simulink model "model_chirp_control_conMR_BoucWen"  (R2021b)
settings: Solver=VariableStepAuto  StartTime=0.0  StopTime=t_final2  FixedStep=tsam  RelTol=1e-3  EnableMultiTasking=on
values from neighbouring files (symbols this model uses):
  A = [      0          1       0    0      0    0 ... (first row only)    [model.m]
  I1 = 0.01    [Run_MdE_Research_Report_con_MR_damper.m]
  kt = ((2*pi*ft)^2)*mt    [Run_MdE_Research_Report.m]    (also in Run_MdE_Research_Report_con_MR_damper.m; my_script.m)
  mt = mu*m1    (= 0.02)    [Run_MdE_Research_Report.m]    (also in Run_MdE_Research_Report_con_MR_damper.m = 40; my_script.m)
undefined symbols (not defined in the file or in its folder): B, C, D_Gs, k0, N_Gs, ndata2, t_final2, tsam, x0
libraries: simulink x1
settings Model: Creator=user  LastModifiedBy=luismiguelmartinezgomez
settings SolverCC: AlgebraicLoopSolver=TrustRegion
settings DataIOCC: LimitDataPoints=on  SaveFormat=Array  SignalLoggingSaveFormat=ModelDataLogs  ReturnWorkspaceOutputs=off  SignalLoggingName=sigsOut
settings OptimizationCC: InitFltsAndDblsToZero=on  LifeSpan=inf
settings DebuggingCC: SaveWithParameterizedLinksMsg=none  UnderspecifiedInitializationDetection=Classic  MergeDetectMultiDrivingBlocksExec=none  SignalResolutionControl=TryResolveAllWithWarning  MultiTaskDSMMsg=warning  MultiTaskCondExecSysMsg=none  FcnCallInpInsideContextMsg=warning  SFUnexpectedBacktrackingDiag=warning  SFNoUnconditionalDefaultTransitionDiag=warning  SFMachineParentedDataDiag=warning  ArithmeticOperatorsInVariantConditions=warning
settings HardwareCC: ProdBitPerPointer=32  ProdBitPerSizeT=32  ProdBitPerPtrDiffT=32  ProdLargestAtomicFloat=None  ProdIntDivRoundTo=Undefined  ProdEndianess=Unspecified  ProdWordSize=32  ProdHWDeviceType=32-bit Generic  TargetBitPerLong=64  TargetBitPerPointer=64  TargetBitPerSizeT=64  TargetBitPerPtrDiffT=64  TargetLongLongMode=on  TargetIntDivRoundTo=Zero  TargetEndianess=LittleEndian  TargetWordSize=64  TargetHWDeviceType=MATLAB Host  ProdEqTarget=off
settings ModelReferenceCC: PropagateSignalLabelsOutOfModel=off
settings SFSimCC: SimUseLocalCustomCode=off  CustomCodeUndefinedFunction=UseInterfaceOnly
settings RTWCC: RTWUseLocalCustomCode=off
settings CodeAppCC: StateflowObjectComments=on
settings GRTTargetCC: TargetFcnLib=ansi_tfl_tmw.mat  TargetLangStandard=C89/C90 (ANSI)  CombineOutputUpdateFcns=off  GRTInterface=on
settings ConfigComp: CovMetricSettings=dw  CovSaveCumulativeToWorkspaceVar=on  CovSaveSingleToWorkspaceVar=on  CovExternalEMLEnable=off  CovSFcnEnable=off

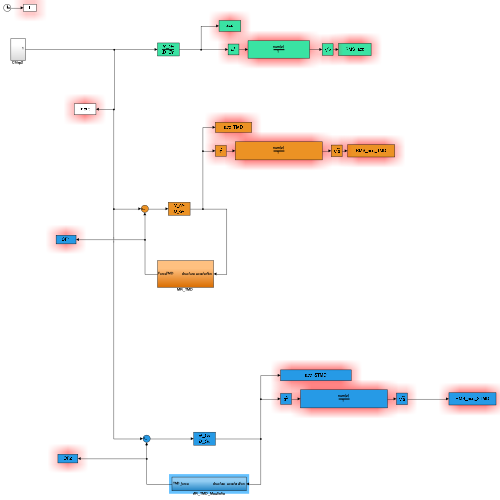
[thumbnail: Simulink's stored preview of the top-level diagram]
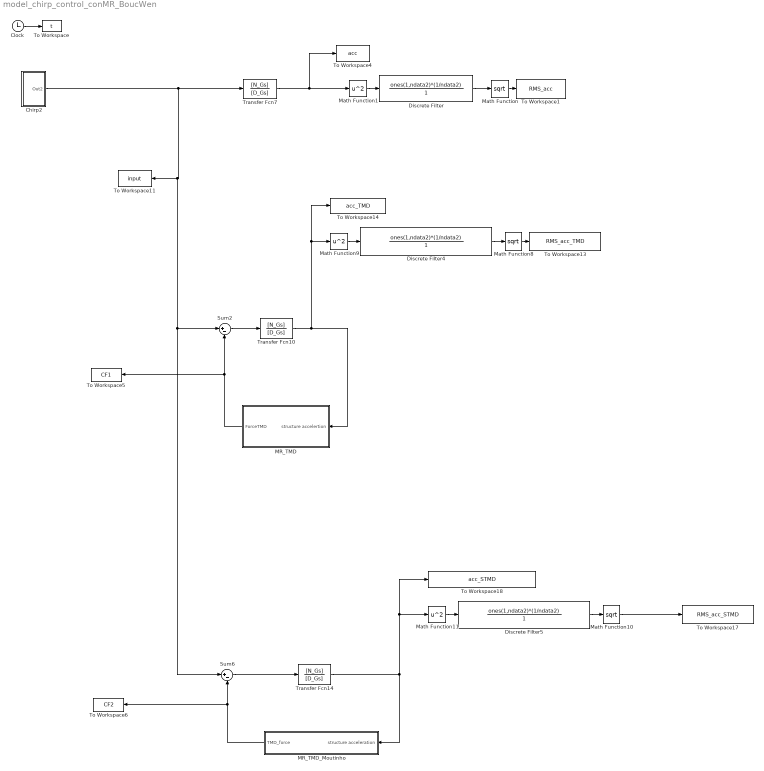
== system model_chirp_control_conMR_BoucWen ==
  Chirp2 : Subsystem
  Clock : Clock
  Discrete Filter : DiscreteFilter  Numerator=ones(1,ndata2)*(1/ndata2)  Denominator=1  SampleTime=tsam
  Discrete Filter4 : DiscreteFilter  Numerator=ones(1,ndata2)*(1/ndata2)  Denominator=1  SampleTime=tsam
  Discrete Filter5 : DiscreteFilter  Numerator=ones(1,ndata2)*(1/ndata2)  Denominator=1  SampleTime=tsam
  MR_TMD : Subsystem
  MR_TMD_Moutinho : Subsystem
  Math Function : Math  Operator=sqrt  SignedPower=on  SampleTime=tsam  SaturateOnIntegerOverflow=on
  Math Function1 : Math  Operator=square  SignedPower=on  SampleTime=tsam  SaturateOnIntegerOverflow=on
  Math Function10 : Math  Operator=sqrt  SignedPower=on  SampleTime=tsam  SaturateOnIntegerOverflow=on
  Math Function11 : Math  Operator=square  SignedPower=on  SampleTime=tsam  SaturateOnIntegerOverflow=on
  Math Function8 : Math  Operator=sqrt  SignedPower=on  SampleTime=tsam  SaturateOnIntegerOverflow=on
  Math Function9 : Math  Operator=square  SignedPower=on  SampleTime=tsam  SaturateOnIntegerOverflow=on
  Sum2 : Sum  Inputs=|+-
  Sum6 : Sum  Inputs=|+-
  To Workspace : ToWorkspace  VariableName=t  SampleTime=tsam
  To Workspace1 : ToWorkspace  VariableName=RMS_acc  SampleTime=tsam
  To Workspace11 : ToWorkspace  VariableName=input  SampleTime=tsam
  To Workspace13 : ToWorkspace  VariableName=RMS_acc_TMD  SampleTime=tsam
  To Workspace14 : ToWorkspace  VariableName=acc_TMD  SampleTime=tsam
  To Workspace17 : ToWorkspace  VariableName=RMS_acc_STMD  SampleTime=tsam
  To Workspace18 : ToWorkspace  VariableName=acc_STMD  SampleTime=tsam
  To Workspace4 : ToWorkspace  VariableName=acc  SampleTime=tsam
  To Workspace5 : ToWorkspace  VariableName=CF1  SampleTime=tsam
  To Workspace6 : ToWorkspace  VariableName=CF2  SampleTime=tsam
  Transfer Fcn10 : TransferFcn  Numerator=[N_Gs]  Denominator=[D_Gs]
  Transfer Fcn14 : TransferFcn  Numerator=[N_Gs]  Denominator=[D_Gs]
  Transfer Fcn7 : TransferFcn  Numerator=[N_Gs]  Denominator=[D_Gs]
  wires:
  Clock/1 -> To Workspace/1
  Math Function1/1 -> Discrete Filter/1
  Discrete Filter/1 -> Math Function/1
  Math Function/1 -> To Workspace1/1
  Sum2/1 -> Transfer Fcn10/1
  Math Function9/1 -> Discrete Filter4/1
  Discrete Filter4/1 -> Math Function8/1
  Math Function8/1 -> To Workspace13/1
  MR_TMD/1(ForceTMD) -> Sum2/2, To Workspace5/1
  Transfer Fcn7/1 -> Math Function1/1, To Workspace4/1
  Transfer Fcn10/1 -> MR_TMD/1(structure accelertion), To Workspace14/1, Math Function9/1
  Math Function11/1 -> Discrete Filter5/1
  Discrete Filter5/1 -> Math Function10/1
  Math Function10/1 -> To Workspace17/1
  Sum6/1 -> Transfer Fcn14/1
  Chirp2/1(Out2) -> Sum2/1, Sum6/1, To Workspace11/1, Transfer Fcn7/1
  Transfer Fcn14/1 -> MR_TMD_Moutinho/1(structure acceleration), Math Function11/1, To Workspace18/1
  MR_TMD_Moutinho/1(TMD_force) -> To Workspace6/1, Sum6/2

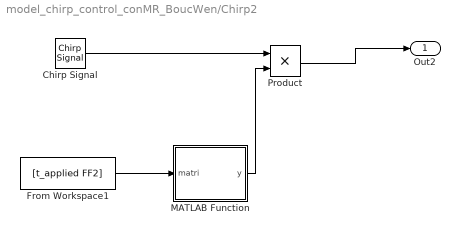
== system model_chirp_control_conMR_BoucWen/Chirp2 ==
  Chirp Signal : simulink/Sources/Chirp Signal  f1=f_ini  T=t_final2  f2=f_fin
  From Workspace1 : FromWorkspace  VariableName=[t_applied FF2]  SampleTime=tsam  ZeroCross=off
  MATLAB Function : MATLAB Function  TreatAsAtomicUnit=on
  Product : Product
  Out2 : Outport
  wires:
  Chirp Signal/1 -> Product/1
  MATLAB Function/1(y) -> Product/2
  Product/1 -> Out2/1
  From Workspace1/1 -> MATLAB Function/1(matri)

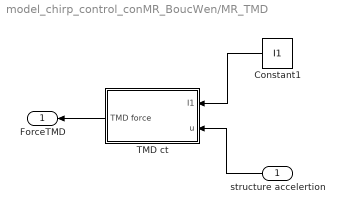
== system model_chirp_control_conMR_BoucWen/MR_TMD ==
  structure accelertion : Inport
  Constant1 : Constant  Value=I1
  TMD ct : Subsystem
  ForceTMD : Outport
  wires:
  TMD ct/1(TMD force) -> ForceTMD/1
  structure accelertion/1 -> TMD ct/2(u)
  Constant1/1 -> TMD ct/1(I1)

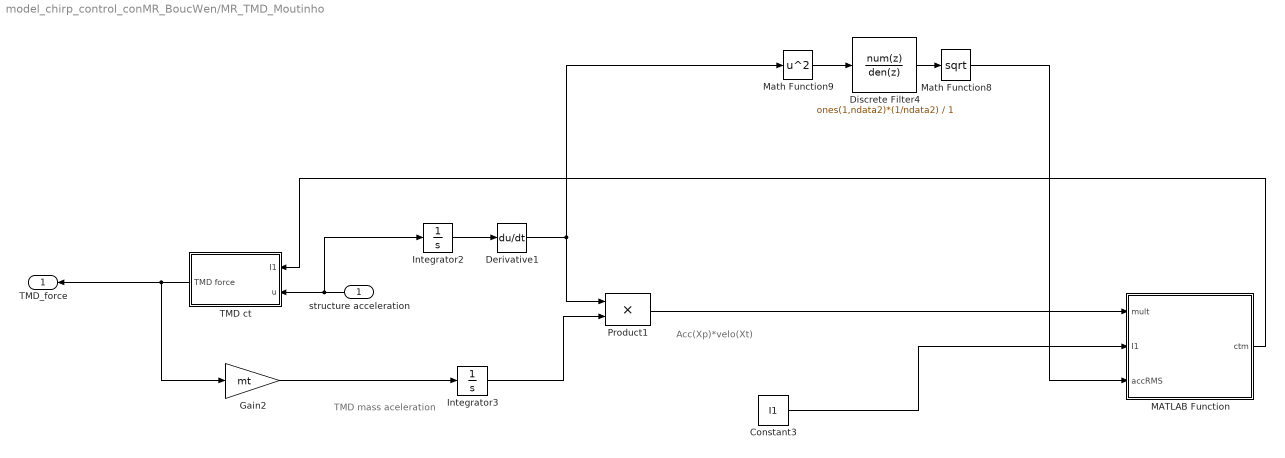
== system model_chirp_control_conMR_BoucWen/MR_TMD_Moutinho ==
  note: TMD mass
      | aceleration
  note: Acc(Xp)*velo(Xt)
  structure acceleration : Inport
  Constant3 : Constant  Value=I1
  Derivative1 : Derivative
  Discrete Filter4 : DiscreteFilter  Numerator=ones(1,ndata2)*(1/ndata2)  Denominator=1  SampleTime=tsam
  Gain2 : Gain  Gain=mt
  Integrator2 : Integrator
  Integrator3 : Integrator
  MATLAB Function : MATLAB Function  TreatAsAtomicUnit=on
  Math Function8 : Math  Operator=sqrt  SignedPower=on  SampleTime=tsam  SaturateOnIntegerOverflow=on
  Math Function9 : Math  Operator=square  SignedPower=on  SampleTime=tsam  SaturateOnIntegerOverflow=on
  Product1 : Product  OutDataTypeStr=double  SaturateOnIntegerOverflow=on
  TMD ct : Subsystem
  TMD_force : Outport
  wires:
  TMD ct/1(TMD force) -> Gain2/1, TMD_force/1
  Integrator3/1 -> Product1/2
  Product1/1 -> MATLAB Function/1(mult)
  MATLAB Function/1(ctm) -> TMD ct/1(I1)
  structure acceleration/1 -> Integrator2/1, TMD ct/2(u)
  Gain2/1 -> Integrator3/1
  Constant3/1 -> MATLAB Function/2(I1)
  Math Function9/1 -> Discrete Filter4/1
  Discrete Filter4/1 -> Math Function8/1
  Math Function8/1 -> MATLAB Function/3(accRMS)
  Integrator2/1 -> Derivative1/1
  Derivative1/1 -> Product1/1, Math Function9/1

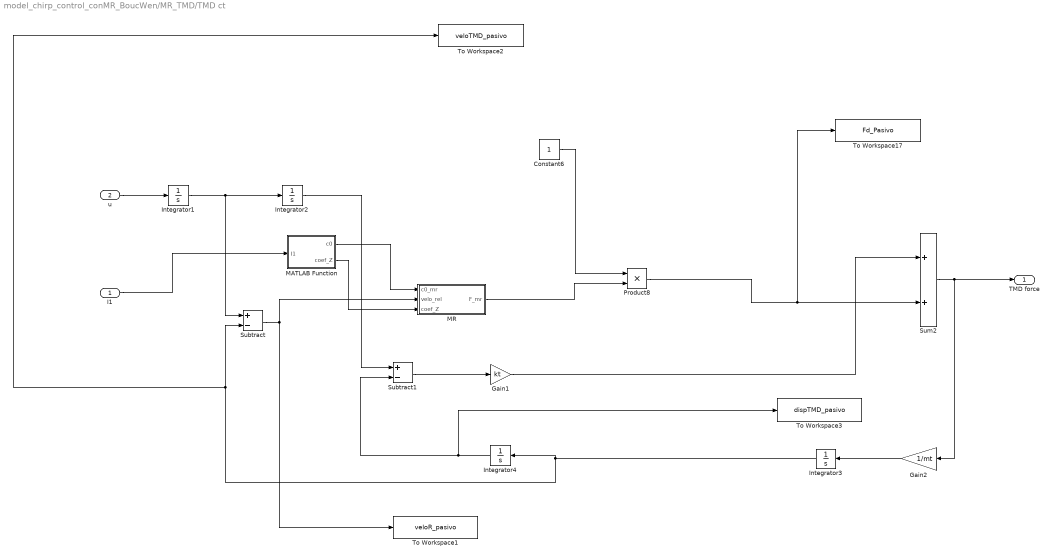
== system model_chirp_control_conMR_BoucWen/MR_TMD/TMD ct ==
  I1 : Inport
  u : Inport  Port=2
  Constant6 : Constant
  Gain1 : Gain  Gain=kt
  Gain2 : Gain  Gain=1/mt
  Integrator{1..4} (4 alike) : Integrator
  MATLAB Function : MATLAB Function  TreatAsAtomicUnit=on
  MR : Subsystem
  Product8 : Product
  Subtract : Sum  Inputs=+-
  Subtract1 : Sum  Inputs=+-
  Sum2 : Sum
  To Workspace1 : ToWorkspace  VariableName=veloR_pasivo  SampleTime=tsam
  To Workspace17 : ToWorkspace  VariableName=Fd_Pasivo  SampleTime=tsam
  To Workspace2 : ToWorkspace  VariableName=veloTMD_pasivo  SampleTime=tsam
  To Workspace3 : ToWorkspace  VariableName=dispTMD_pasivo  SampleTime=tsam
  TMD force : Outport
  wires:
  Integrator1/1 -> Subtract/1, Integrator2/1
  u/1 -> Integrator1/1
  I1/1 -> MATLAB Function/1(I1)
  Integrator3/1 -> Integrator4/1, To Workspace2/1, Subtract/2
  Subtract/1 -> MR/2(velo_rel), To Workspace1/1
  Gain2/1 -> Integrator3/1
  Integrator4/1 -> To Workspace3/1, Subtract1/2
  Integrator2/1 -> Subtract1/1
  Subtract1/1 -> Gain1/1
  Gain1/1 -> Sum2/1
  Sum2/1 -> Gain2/1, TMD force/1
  MATLAB Function/1(c0) -> MR/1(c0_mr)
  MATLAB Function/2(coef_Z) -> MR/3(coef_Z)
  Constant6/1 -> Product8/1
  MR/1(F_mr) -> Product8/2
  Product8/1 -> To Workspace17/1, Sum2/2

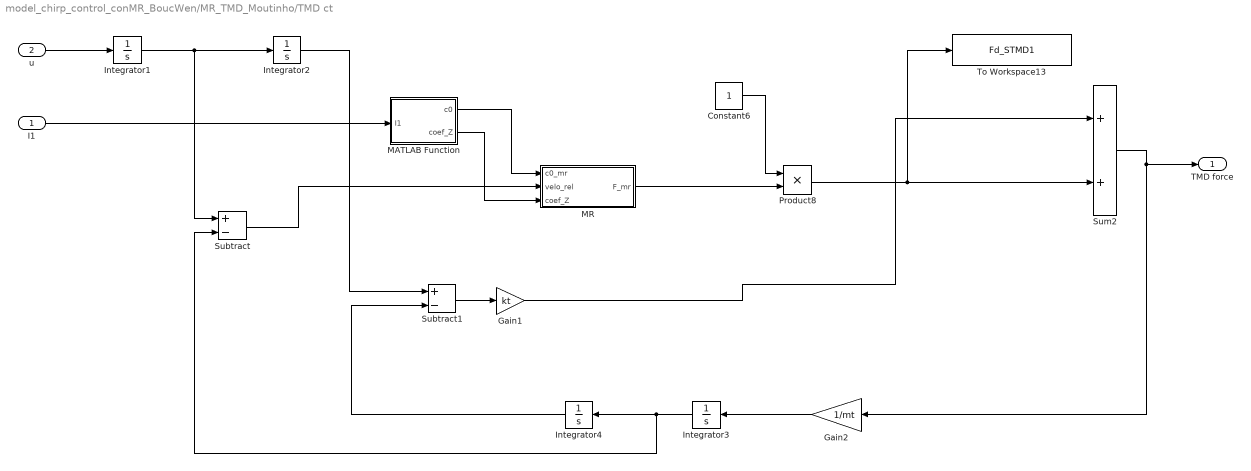
== system model_chirp_control_conMR_BoucWen/MR_TMD_Moutinho/TMD ct ==
  I1 : Inport
  u : Inport  Port=2
  Constant6 : Constant
  Gain1 : Gain  Gain=kt
  Gain2 : Gain  Gain=1/mt
  Integrator{1..4} (4 alike) : Integrator
  MATLAB Function : MATLAB Function  TreatAsAtomicUnit=on
  MR : Subsystem
  Product8 : Product
  Subtract : Sum  Inputs=+-
  Subtract1 : Sum  Inputs=+-
  Sum2 : Sum
  To Workspace13 : ToWorkspace  VariableName=Fd_STMD1  SampleTime=tsam
  TMD force : Outport
  wires:
  Integrator1/1 -> Subtract/1, Integrator2/1
  u/1 -> Integrator1/1
  Integrator3/1 -> Integrator4/1, Subtract/2
  Gain2/1 -> Integrator3/1
  Integrator4/1 -> Subtract1/2
  Integrator2/1 -> Subtract1/1
  Subtract1/1 -> Gain1/1
  Gain1/1 -> Sum2/1
  Sum2/1 -> Gain2/1, TMD force/1
  I1/1 -> MATLAB Function/1(I1)
  Subtract/1 -> MR/2(velo_rel)
  MATLAB Function/1(c0) -> MR/1(c0_mr)
  MATLAB Function/2(coef_Z) -> MR/3(coef_Z)
  Constant6/1 -> Product8/1
  MR/1(F_mr) -> Product8/2
  Product8/1 -> To Workspace13/1, Sum2/2

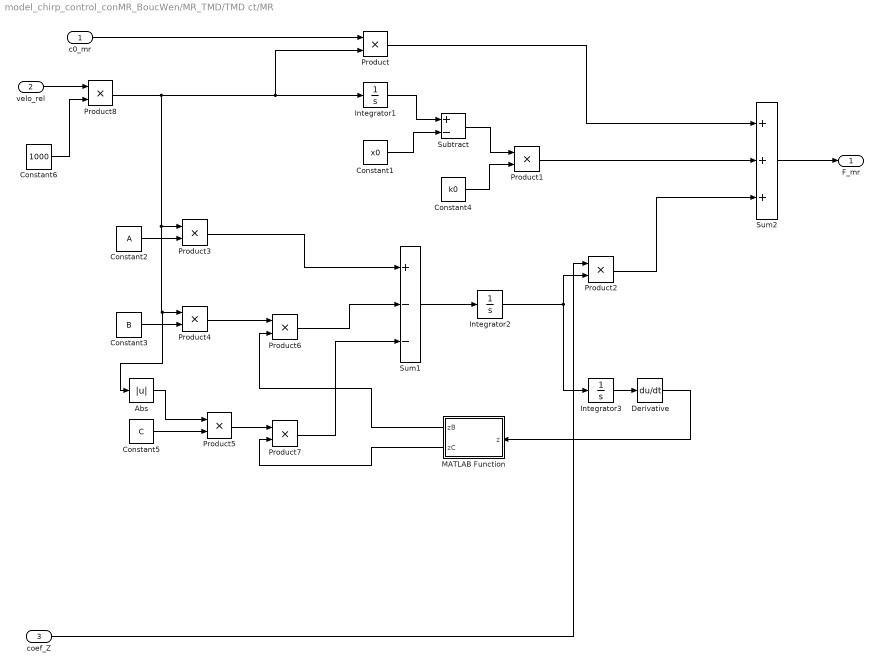
== system model_chirp_control_conMR_BoucWen/MR_TMD/TMD ct/MR ==
  c0_mr : Inport
  velo_rel : Inport  Port=2
  coef_Z : Inport  Port=3
  Abs : Abs
  Constant1 : Constant  Value=x0
  Constant2 : Constant  Value=A
  Constant3 : Constant  Value=B
  Constant4 : Constant  Value=k0
  Constant5 : Constant  Value=C
  Constant6 : Constant  Value=1000
  Derivative : Derivative
  Integrator1 : Integrator
  Integrator2 : Integrator  UpperSaturationLimit=1  LowerSaturationLimit=-1
  Integrator3 : Integrator
  MATLAB Function : MATLAB Function  TreatAsAtomicUnit=on
  Product{,1..8} (9 alike) : Product
  Subtract : Sum  Inputs=+-
  Sum1 : Sum  Inputs=+--
  Sum2 : Sum  Inputs=+++
  F_mr : Outport
  wires:
  c0_mr/1 -> Product/1
  Integrator1/1 -> Subtract/1
  Constant1/1 -> Subtract/2
  Subtract/1 -> Product1/1
  Constant4/1 -> Product1/2
  Sum2/1 -> F_mr/1
  Product1/1 -> Sum2/2
  Product/1 -> Sum2/1
  coef_Z/1 -> Product2/1
  Integrator2/1 -> Integrator3/1, Product2/2
  Constant2/1 -> Product3/2
  Constant3/1 -> Product4/2
  Constant5/1 -> Product5/2
  Sum1/1 -> Integrator2/1
  Product3/1 -> Sum1/1
  Product4/1 -> Product6/1
  Product5/1 -> Product7/1
  MATLAB Function/1(zB) -> Product6/2
  Product6/1 -> Sum1/2
  MATLAB Function/2(zC) -> Product7/2
  Product7/1 -> Sum1/3
  Product2/1 -> Sum2/3
  Integrator3/1 -> Derivative/1
  Derivative/1 -> MATLAB Function/1(z)
  Abs/1 -> Product5/1
  Product8/1 -> Product3/1, Abs/1, Product4/1, Integrator1/1, Product/2
  velo_rel/1 -> Product8/1
  Constant6/1 -> Product8/2

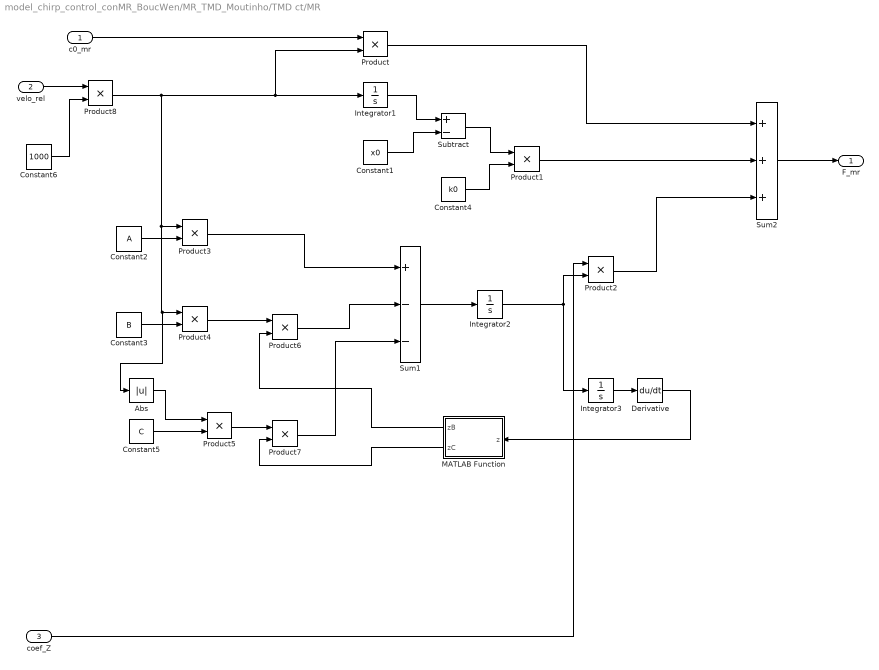
== system model_chirp_control_conMR_BoucWen/MR_TMD_Moutinho/TMD ct/MR ==
  c0_mr : Inport
  velo_rel : Inport  Port=2
  coef_Z : Inport  Port=3
  Abs : Abs
  Constant1 : Constant  Value=x0
  Constant2 : Constant  Value=A
  Constant3 : Constant  Value=B
  Constant4 : Constant  Value=k0
  Constant5 : Constant  Value=C
  Constant6 : Constant  Value=1000
  Derivative : Derivative
  Integrator1 : Integrator
  Integrator2 : Integrator  UpperSaturationLimit=1  LowerSaturationLimit=-1
  Integrator3 : Integrator
  MATLAB Function : MATLAB Function  TreatAsAtomicUnit=on
  Product{,1..8} (9 alike) : Product
  Subtract : Sum  Inputs=+-
  Sum1 : Sum  Inputs=+--
  Sum2 : Sum  Inputs=+++
  F_mr : Outport
  wires:
  c0_mr/1 -> Product/1
  Integrator1/1 -> Subtract/1
  Constant1/1 -> Subtract/2
  Subtract/1 -> Product1/1
  Constant4/1 -> Product1/2
  Sum2/1 -> F_mr/1
  Product1/1 -> Sum2/2
  Product/1 -> Sum2/1
  coef_Z/1 -> Product2/1
  Integrator2/1 -> Integrator3/1, Product2/2
  Constant2/1 -> Product3/2
  Constant3/1 -> Product4/2
  Constant5/1 -> Product5/2
  Sum1/1 -> Integrator2/1
  Product3/1 -> Sum1/1
  Product4/1 -> Product6/1
  Product5/1 -> Product7/1
  MATLAB Function/1(zB) -> Product6/2
  Product6/1 -> Sum1/2
  MATLAB Function/2(zC) -> Product7/2
  Product7/1 -> Sum1/3
  Product2/1 -> Sum2/3
  Integrator3/1 -> Derivative/1
  Derivative/1 -> MATLAB Function/1(z)
  Abs/1 -> Product5/1
  Product8/1 -> Product3/1, Abs/1, Product4/1, Integrator1/1, Product/2
  velo_rel/1 -> Product8/1
  Constant6/1 -> Product8/2

== matlab function model_chirp_control_conMR_BoucWen/MR_TMD/TMD ct/MR/MATLAB Function ==
  data: z input; zB output; zC output
function [zB,zC] = fcn(z)
n = 1;
zB = abs(z)^n;
zC = z*abs(z)^(n-1);

== matlab function model_chirp_control_conMR_BoucWen/MR_TMD/TMD ct/MATLAB Function ==
  data: I1 input; c0 output; coef_Z output
function [c0,coef_Z] = fcn(I1)
coef_Z = -9.66*I1^3 + 9.76*I1^2 + 1.12*I1 + 0.10;
c0 = 4.48*I1^4 - 4.74*I1^3 + 1.35*I1^2 + 0.05*I1 + 0.01;

== matlab function model_chirp_control_conMR_BoucWen/Chirp2/MATLAB Function ==
  data: y output; matri input
function y = fcn(matri)

% time = matri(:,1);
% force = matri(:,2);
% 
% pos = find( u>= time);
% pos2 = pos(1);


y = matri; %force(pos);

== matlab function model_chirp_control_conMR_BoucWen/MR_TMD_Moutinho/MATLAB Function ==
  data: mult input; ctm output; I1 input; accRMS input
function ctm = fcn(mult,I1,accRMS)
    % Semi-active trigger
    if accRMS > 0.05
        if mult <= 0
            ctm = I1;
        else
            ctm = 0.5;
        end
    else
        ctm = I1;
    end
end

== matlab function model_chirp_control_conMR_BoucWen/MR_TMD_Moutinho/TMD ct/MATLAB Function ==
  data: I1 input; c0 output; coef_Z output
function [c0,coef_Z] = fcn(I1)
coef_Z = -9.66*I1^3 + 9.76*I1^2 + 1.12*I1 + 0.10;
c0 = 4.48*I1^4 - 4.74*I1^3 + 1.35*I1^2 + 0.05*I1 + 0.01;

== matlab function model_chirp_control_conMR_BoucWen/MR_TMD_Moutinho/TMD ct/MR/MATLAB Function ==
  data: z input; zB output; zC output
function [zB,zC] = fcn(z)
n = 1;
zB = abs(z)^n;
zC = z*abs(z)^(n-1);
